simulink model "HITL_Development_Model"  (R2022a)
settings: Solver=VariableStepAuto  StartTime=0.0  StopTime=10.0  RelTol=1e-3
StartFcn:
  | startFunc()
values from neighbouring files (symbols this model uses):
  CG0 = readmatrix("Inertial Props.xlsx",'Sheet','Static Line Items','Range','U3:W3')    [startFunc.m]
  I0 = readmatrix("Inertial Props.xlsx",'Sheet','Static Line Items','Range','U7:W9')    [startFunc.m]
  M0 = readmatrix("Inertial Props.xlsx",'Sheet','Static Line Items','Range','T1:T1')    [startFunc.m]
libraries: shared6dof x1
settings Model: Creator=natha  LastModifiedBy=natha

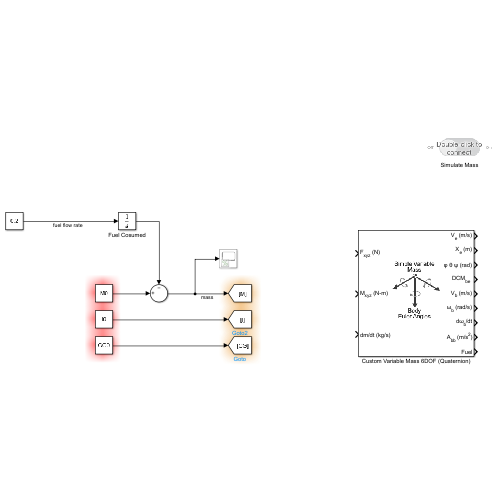
[thumbnail: Simulink's stored preview of the top-level diagram]
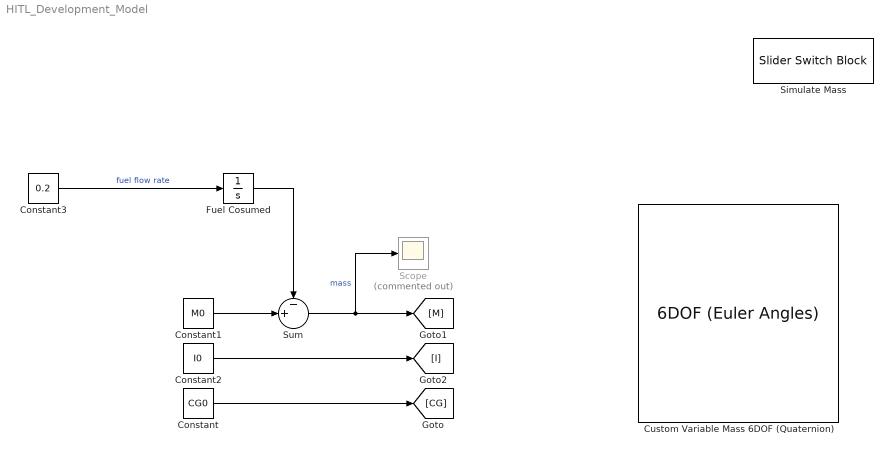
== system HITL_Development_Model ==
  Constant : Constant  Value=CG0
  Constant1 : Constant  Value=M0
  Constant2 : Constant  Value=I0
  Constant3 : Constant  Value=0.2
  Custom Variable Mass 6DOF (Quaternion) : shared6dof/6DOF (Euler Angles)  units=Metric (MKS)  mtype=Simple Variable  rep=Euler Angles  xme_0=[0 0 0]  Vm_0=[0 0 0]  eul_0=[0 0 0]  pm_0=[0 0 0]  mass_0=1.0  mass_e=0.5  mass_f=2.0  inertia=eye(3)  inertia_e=eye(3)  inertia_f=2*eye(3)  k_quat=1.0  vre_flag=off  abi_flag=off  aMode=0  xme_statename=''  Vm_statename=''  eul_statename=''  quat_statename=''  pm_statename=''  mass_statename=''
      settings: SourceProductBaseCode=AE,PW,DR,MT,VE
  Fuel Cosumed : Integrator
  Scope : Scope  Commented=on
  Simulate Mass : SliderSwitchBlock
      settings: Values={{'Off', 'On'}, [0 1]}
  Sum : Sum  Inputs=-+|
  wires:
  Constant/1 -> [CG]
  Constant1/1 -> Sum/2
  Constant2/1 -> [I]
  Sum/1 -> Scope/1, [M]  "mass"
  Fuel Cosumed/1 -> Sum/1
  Constant3/1 -> Fuel Cosumed/1  "fuel flow rate"
